simulink model "Pravahan_Powertrain_Powertrnblkset"  (R2023a)
settings: Solver=VariableStepAuto  StartTime=0.0  StopTime=5856  RelTol=1e-3
model workspace (MAT data in the model file):
  RPM = [0; 500; 500; 500; 500; 1000; 2000; 3000; 4000; 3000; 3000; 3000; 3000; 3300; 3300; 3300; 3000; 3000; 3000; 3000; 3000; 3500; 3500; 3500; 3500; 3000; 3000; 3000; 2500; 2000; 0; 0; 500; 1000; 2000; 3000; 4000; 3000; 3000; 3000; 3000; 3300; 3300; 3300; 3000; 3000; 3000; 3000; 3000; 3500; 3500; 3500; 3500; 3000; 3000; 3000; 3000; 3000; 3000; 2500; 2000; 0]
  Time = [0; 96; 192; 288; 384; 480; 576; 672; 768; 864; 960; 1056; 1152; 1248; 1344; 1440; 1536; 1632; 1728; 1824; 1920; 2016; 2112; 2208; 2304; 2400; 2496; 2592; 2688; 2784; 2880; 2976; 3072; 3168; 3264; 3360; 3456; 3552; 3648; 3744; 3840; 3936; 4032; 4128; 4224; 4320; 4416; 4512; 4608; 4704; 4800; 4896; 4992; 5088; 5184; 5280; 5376; 5472; 5568; 5664; 5760; 5856]
libraries: autolibrcnetworksystem x1, autolibmappedmotor x1
settings Model: Creator=Abhinandan  LastModifiedBy=Abhinandan

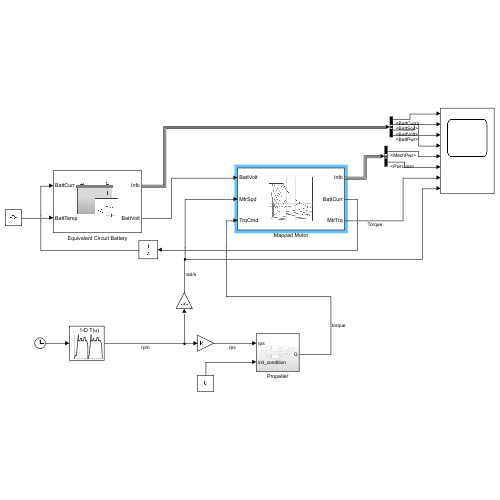
[thumbnail: Simulink's stored preview of the top-level diagram]
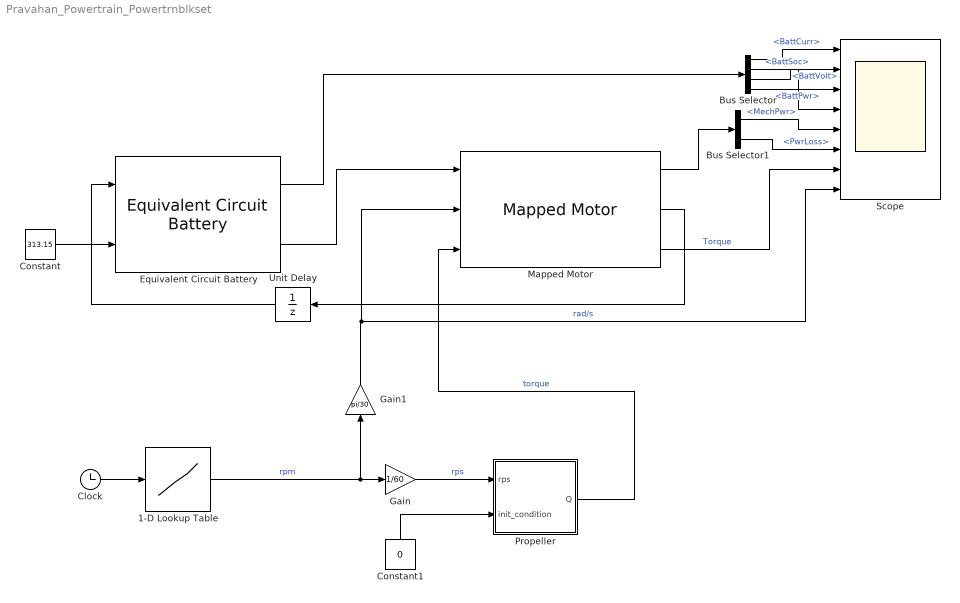
== system Pravahan_Powertrain_Powertrnblkset ==
  1-D Lookup Table : Lookup_n-D  NumberOfTableDimensions=1  BreakpointsForDimension1=Time  Table=RPM  InternalRulePriority=Speed  RndMeth=Simplest
  Bus Selector : BusSelector  OutputSignals=BattCurr,BattSoc,BattVolt,BattPwr
  Bus Selector1 : BusSelector  OutputSignals=MechPwr,PwrLoss
  Clock : Clock
  Constant : Constant  Value=313.15
  Constant1 : Constant  Value=0
  Equivalent Circuit Battery : autolibrcnetworksystem/Equivalent Circuit Battery  CapacityCtrl=Parameter  OutputVlt=Unfiltered  NumRC=1  Em=|  R0=|  SOC_BP=|  Temperature_BP=[293.15 313.15]  BattCap=[350 350]  BattCapInit=297.5  InitialCapVoltage=0  Tc=1/1000  Vinit=4.193  R1=|  C1=|  R2=|  C2=|  R3=|  C3=|  R4=|  C4=|  R5=|  C5=|  Vu=Inf  Vl=-Inf  RefBlkName='autolibrcnetworksystem/Equivalent Circuit Battery'
      Em=|
      | 62*[3.5042 3.5136;
      | 3.5573 3.5646;
      | 3.6009 3.6153;
      | 3.6393 3.6565;
      | 3.6742 3.6889;
      | 3.7121 3.7214;
      | 3.7937 3.8078;
      | 3.8753 3.8945;
      | 3.97 3.9859;
      | 4.0764 4.0821;
      | 4.1924 4.193]
      R0=|
      | (62/14)*[0.011448 0.0090006;
      | 0.011038 0.0089655;
      | 0.011281 0.0091261;
      | 0.011236 0.0091099;
      | 0.010959 0.008957;
      | 0.010714 0.0087969;
      | 0.010698 0.0089126;
      | 0.010712 0.0090517;
      | 0.010917 0.0090444;
      | 0.011304 0.0088992;
      | 0.011603 0.0089015
      | ]
      SOC_BP=|
      | [0
      | 0.1
      | 0.2
      | 0.3
      | 0.4
      | 0.5
      | 0.6
      | 0.7
      | 0.8
      | 0.9
      | 1]
      R1=|
      | (62/14)*[0.010342 0.0012244;
      | 0.0067316 0.0011396;
      | 0.0051156 0.0012661;
      | 0.0043447 0.0012265;
      | 0.0038826 0.0011163;
      | 0.0034226 0.0009968;
      | 0.003346 0.0011458;
      | 0.0033222 0.001345;
      | 0.0033201 0.0013091;
      | 0.0032886 0.0010986;
      | 0.0028114 0.0010309]
      C1=|
      | (14/62)*[2287.7 11897;
      | 6122 24515;
      | 18460 42098;
      | 20975 44453;
      | 15254 33098;
      | 10440 24492;
      | 13903 32975;
      | 16694 40007;
      | 15784 35937;
      | 12165 26430;
      | 9118 24795]
      R2=|
      | [0.010342 0.0012244;
      | 0.0067316 0.0011396;
      | 0.0051156 0.0012661;
      | 0.0043447 0.0012265;
      | 0.0038826 0.0011163;
      | 0.0034226 0.0009968;
      | 0.003346 0.0011458;
      | 0.0033222 0.001345;
      | 0.0033201 0.0013091;
      | 0.0032886 0.0010986;
      | 0.0028114 0.0010309]
      C2=|
      | [2287.7 11897;
      | 6122 24515;
      | 18460 42098;
      | 20975 44453;
      | 15254 33098;
      | 10440 24492;
      | 13903 32975;
      | 16694 40007;
      | 15784 35937;
      | 12165 26430;
      | 9118 24795]
      R3=|
      | [0.010342 0.0012244;
      | 0.0067316 0.0011396;
      | 0.0051156 0.0012661;
      | 0.0043447 0.0012265;
      | 0.0038826 0.0011163;
      | 0.0034226 0.0009968;
      | 0.003346 0.0011458;
      | 0.0033222 0.001345;
      | 0.0033201 0.0013091;
      | 0.0032886 0.0010986;
      | 0.0028114 0.0010309]
      C3=|
      | [2287.7 11897;
      | 6122 24515;
      | 18460 42098;
      | 20975 44453;
      | 15254 33098;
      | 10440 24492;
      | 13903 32975;
      | 16694 40007;
      | 15784 35937;
      | 12165 26430;
      | 9118 24795]
      R4=|
      | [0.010342 0.0012244;
      | 0.0067316 0.0011396;
      | 0.0051156 0.0012661;
      | 0.0043447 0.0012265;
      | 0.0038826 0.0011163;
      | 0.0034226 0.0009968;
      | 0.003346 0.0011458;
      | 0.0033222 0.001345;
      | 0.0033201 0.0013091;
      | 0.0032886 0.0010986;
      | 0.0028114 0.0010309]
      C4=|
      | [2287.7 11897;
      | 6122 24515;
      | 18460 42098;
      | 20975 44453;
      | 15254 33098;
      | 10440 24492;
      | 13903 32975;
      | 16694 40007;
      | 15784 35937;
      | 12165 26430;
      | 9118 24795]
      R5=|
      | [0.010342 0.0012244;
      | 0.0067316 0.0011396;
      | 0.0051156 0.0012661;
      | 0.0043447 0.0012265;
      | 0.0038826 0.0011163;
      | 0.0034226 0.0009968;
      | 0.003346 0.0011458;
      | 0.0033222 0.001345;
      | 0.0033201 0.0013091;
      | 0.0032886 0.0010986;
      | 0.0028114 0.0010309]
      C5=|
      | [2287.7 11897;
      | 6122 24515;
      | 18460 42098;
      | 20975 44453;
      | 15254 33098;
      | 10440 24492;
      | 13903 32975;
      | 16694 40007;
      | 15784 35937;
      | 12165 26430;
      | 9118 24795]
  Gain : Gain  Gain=1/60
  Gain1 : Gain  Gain=pi/30
  Mapped Motor : autolibmappedmotor/Mapped Motor  port_config=Speed  param_by=Maximum torque and power  w_t=[ 0 375 750 800 ]  T_t=[0.09 0.08 0.07 0]  torque_max=240  power_max=100000  Tc=0.02  param_loss=Tabulated efficiency data  eff=100  w_eff=375  T_eff=0.08  Piron=0  Pbase=0  w_eff_bp=[-300 -100 0 100 300]  T_eff_bp=[0 80 200 250]  Temp_eff_bp=[233.15 293.15 373.15]  losses_table=[1.49 1.67 2.21 3.10; 0.42 0.69 1.14 2.03; 0.06 0.24 0.78 1.68; 0.42 0.69 1.14 2.03; 1.49 1.67 2.21 3.10]  losses_table_3d=cat(3,[1.49 1.67 2.21 3.10; 0.42 0.69 1.14 2.03; 0.06 0.24 0.78 1.68; 0.42 0.69 1.14 2.03; 1.49 1.67 2.21 3.10],[1.49 1.67 2.21 3.10; 0.42 0.69 1.14 2.03; 0.06 0.24 0.78 1.68; 0.42 0.69 1.14 2.03; 1.49 1.67 2.21 3.10],[1.49 1.67 2.21 3.10; 0.42 0.69 1.14 2.03; 0.06 0.24 0.78 1.68; 0.42 0.69 1.14 2.03; 1.49 1.67 2.21 3.10])  efficiency_table=[94 94 94 94; 94 94 94 94; 94 94 94 94; 94 94 94 94; 94 94 94 94]  efficiency_table_3d=cat(3,[95 95 95 95; 95 95 95 95; 95 95 95 95; 95 95 95 95; 95 95 95 95],[95 95 95 95; 95 95 95 95; 95 95 95 95; 95 95 95 95; 95 95 95 95],[95 95 95 95; 95 95 95 95; 95 95 95 95; 95 95 95 95; 95 95 95 95])  J=5e-6  b=1e-5  omega_o=0  T_t_extended=[0 0.07 0.08 0.09 0.08 0.07 0]  w_t_extended=[-800 -750 -375 0 375 750 800]  KLossIron=0  KLossCopper=0  x_w_eff_vec=[-300 -100 0 100 300]  x_T_eff_vec=[-250 -200 -80 0 80 200 250]  x_tmp_eff_vec=[-0.09 -0.06 -0.03 0 0.03 0.06 0.09]  x_losses_mat=[4787.23404255319 3829.78723404255 1531.91489361702 0 1440 3600 4500;1595.74468085106 1276.59574468085 510.63829787234 0 480 1200 1500;0 0 0 0 0 0 0;1500 1200 480 0 510.63829787234 1276.59574468085 1595.74468085106;4500 3600 1440 0 1531.91489361702 3829.78723404255 4787.23404255319]  x_losses_mat_3d=[37.8947368421052 25.2631578947368 12.6315789473684 0 12 24 36;18.9473684210526 12.6315789473684 6.3157894736842 0 5.99999999999999 12 18;0 0 0 0 0 0 0;18 12 5.99999999999999 0 6.3157894736842 12.6315789473684 18.9473684210526;36 24 12 0 12.6315789473684 25.2631578947368 37.8947368421052]  CalLossMapData={}  CalLossWithTempMapData={}  aMode=1  RefBlkName='autolibmappedmotor/Mapped Motor'
      settings: LibrarySourceBlock=autolibemachines/Mapped Motor
  Propeller : Subsystem
  Scope : Scope  NumInputPorts=8
  Unit Delay : UnitDelay  SampleTime=-1  HasFrameUpgradeWarning=on
  wires:
  Equivalent Circuit Battery/2 -> Mapped Motor/1
  Equivalent Circuit Battery/1 -> Bus Selector/1
  Mapped Motor/2 -> Unit Delay/1
  Mapped Motor/1 -> Bus Selector1/1
  Constant/1 -> Equivalent Circuit Battery/2
  Bus Selector/1 -> Scope/1  "<BattCurr>"
  Bus Selector/2 -> Scope/4  "<BattSoc>"
  Bus Selector/3 -> Scope/2  "<BattVolt>"
  Bus Selector/4 -> Scope/3  "<BattPwr>"
  Bus Selector1/1 -> Scope/5  "<MechPwr>"
  Bus Selector1/2 -> Scope/6  "<PwrLoss>"
  Mapped Motor/3 -> Scope/7  "Torque"
  1-D Lookup Table/1 -> Gain/1, Gain1/1  "rpm"
  Propeller/1(Q) -> Mapped Motor/3  "torque"
  Gain/1 -> Propeller/1(rps)  "rps"
  Constant1/1 -> Propeller/2(init_condition)
  Gain1/1 -> Mapped Motor/2, Scope/8  "rad/s"
  Clock/1 -> 1-D Lookup Table/1
  Unit Delay/1 -> Equivalent Circuit Battery/1

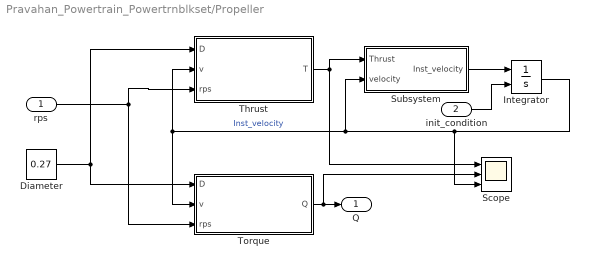
== system Pravahan_Powertrain_Powertrnblkset/Propeller ==
  rps : Inport
  init_condition : Inport  Port=2
  Diameter : Constant  Value=0.27
  Integrator : Integrator  InitialConditionSource=external
  Scope : Scope  NumInputPorts=3
  Subsystem : Subsystem
  Thrust : Subsystem
  Torque : Subsystem
  Q : Outport
  wires:
  Diameter/1 -> Torque/1(D), Thrust/1(D)
  rps/1 -> Torque/3(rps), Thrust/3(rps)
  Thrust/1(T) -> Scope/1, Subsystem/1(Thrust)
  Torque/1(Q) -> Scope/2, Q/1
  Integrator/1 -> Scope/3, Subsystem/2(velocity), Torque/2(v), Thrust/2(v)  "Inst_velocity"
  Subsystem/1(Inst_velocity) -> Integrator/1
  init_condition/1 -> Integrator/2

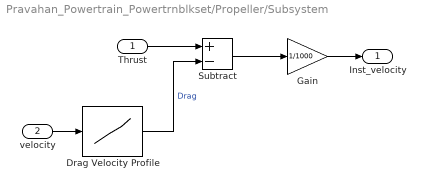
== system Pravahan_Powertrain_Powertrnblkset/Propeller/Subsystem ==
  Thrust : Inport
  velocity : Inport  Port=2
  Drag Velocity Profile : Lookup_n-D  NumberOfTableDimensions=1  BreakpointsForDimension1=[0 2.338181818 4.676363636 7.014545455 8.692839942 8.848719191 11.69090909 14.02909091 16.36727273 18.70545455 21.04363636]  Table=[0.1 2401.65157 3164.117316 3385.663625 3683.299572 1921.181996 1667.962675 1568.170036 1832.926016 1978.032659 2280.974598]  InternalRulePriority=Speed  RndMeth=Simplest
  Gain : Gain  Gain=1/1000
  Subtract : Sum  Inputs=+-
  Inst_velocity : Outport
  wires:
  Thrust/1 -> Subtract/1
  Drag Velocity Profile/1 -> Subtract/2  "Drag"
  Subtract/1 -> Gain/1
  velocity/1 -> Drag Velocity Profile/1
  Gain/1 -> Inst_velocity/1

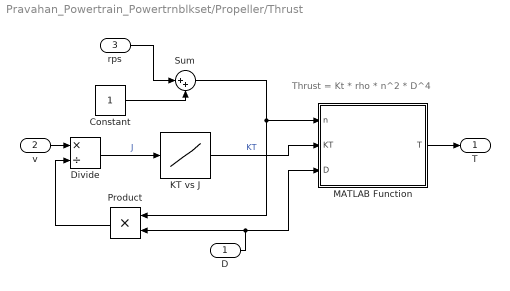
== system Pravahan_Powertrain_Powertrnblkset/Propeller/Thrust ==
  note: Thrust = Kt * rho * n^2 * D^4
  D : Inport
  v : Inport  Port=2
  rps : Inport  Port=3
  Constant : Constant
  Divide : Product  Inputs=*/
  KT vs J : Lookup_n-D  NumberOfTableDimensions=1  BreakpointsForDimension1=[0.0014;0.018198;0.034996;0.053193;0.074191;0.095188;0.109186;0.130184;0.151181;0.172178;0.195976;0.214173;0.23937;0.253368;0.274366;0.295363;0.31916;0.337358;0.354156;0.376553;0.393351;0.411549;0.432546;0.453543;0.473141;0.491339;0.512336;0.533333;0.550131;0.571129;0.589326;0.610324;0.635521;0.652318;0.676115;0.697113;0.72231;0.750306;0.774103;0.7993;0.827297;0.851094;0.869291;0.894488;0.925284;0.953281;0.974278;0.998075;1.019073;1.04147;1.065267;1.093263]  Table=[0.591807;0.582718;0.576664;0.564542;0.55394;0.546373;0.537281;0.531231;0.519112;0.508509;0.496392;0.481235;0.473672;0.466098;0.453978;0.443376;0.431259;0.420654;0.413082;0.397929;0.387323;0.378236;0.367633;0.352479;0.34491;0.332788;0.322185;0.310066;0.296425;0.28734;0.276735;0.264615;0.254017;0.241893;0.228259;0.216139;0.200989;0.185841;0.170689;0.155538;0.144942;0.128273;0.114633;0.102518;0.087372;0.072224;0.061622;0.049505;0.03435;0.026784;0.016185;0.001037]  InterpMethod=Cubic spline
  MATLAB Function : MATLAB Function  TreatAsAtomicUnit=on
  Product : Product
  Sum : Sum  Inputs=|++
  T : Outport
  wires:
  Sum/1 -> Product/1, MATLAB Function/1(n)
  D/1 -> Product/2, MATLAB Function/3(D)
  v/1 -> Divide/1
  Product/1 -> Divide/2
  Divide/1 -> KT vs J/1  "J"
  KT vs J/1 -> MATLAB Function/2(KT)  "KT"
  MATLAB Function/1(T) -> T/1
  rps/1 -> Sum/1
  Constant/1 -> Sum/2

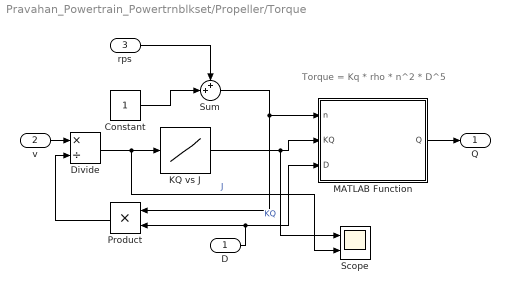
== system Pravahan_Powertrain_Powertrnblkset/Propeller/Torque ==
  note: Torque = Kq * rho * n^2 * D^5
  D : Inport
  v : Inport  Port=2
  rps : Inport  Port=3
  Constant : Constant
  Divide : Product  Inputs=*/
  KQ vs J : Lookup_n-D  NumberOfTableDimensions=1  BreakpointsForDimension1=[0;0.018198;0.039195;0.065792;0.088189;0.111986;0.135783;0.165179;0.188976;0.209974;0.230971;0.261767;0.286964;0.31776;0.338758;0.363955;0.384952;0.410149;0.433946;0.454943;0.47874;0.506737;0.527734;0.548731;0.566929;0.592126;0.620122;0.653718;0.678915;0.706912;0.734908;0.765704;0.7979;0.821697;0.849694;0.874891;0.895888;0.921085;0.940682;0.965879;0.993876;1.019073;1.04287;1.073666;1.096063;1.115661;1.143657;1.164654;1.190833]  Table=[0.096049;0.095151;0.093647;0.092147;0.091252;0.088535;0.087641;0.085232;0.08373;0.081619;0.080115;0.078618;0.07651;0.074102;0.07199;0.069577;0.068074;0.065661;0.063552;0.06144;0.059634;0.057528;0.056024;0.053912;0.051495;0.049994;0.046976;0.044874;0.042461;0.040355;0.037337;0.034928;0.032825;0.030412;0.028305;0.026805;0.024389;0.02228;0.020776;0.018971;0.016865;0.015364;0.013862;0.011758;0.010255;0.008751;0.005732;0.003317;0]
  MATLAB Function : MATLAB Function  TreatAsAtomicUnit=on
  Product : Product
  Scope : Scope  NumInputPorts=2
  Sum : Sum  Inputs=++|
  Q : Outport
  wires:
  MATLAB Function/1(Q) -> Q/1
  D/1 -> Product/2, MATLAB Function/3(D)
  Divide/1 -> Scope/2, KQ vs J/1  "J"
  v/1 -> Divide/1
  KQ vs J/1 -> Scope/1, MATLAB Function/2(KQ)  "KQ"
  Product/1 -> Divide/2
  Sum/1 -> Product/1, MATLAB Function/1(n)
  rps/1 -> Sum/1
  Constant/1 -> Sum/2

== matlab function Pravahan_Powertrain_Powertrnblkset/Propeller/Thrust/MATLAB Function ==
  data: n input; T output; KT input; D input
function T = fcn(n,KT,D)
    rho = 997;
    for i = length(n)
        T = KT * rho * n(i)^2 * D^4;
    end
end

== matlab function Pravahan_Powertrain_Powertrnblkset/Propeller/Torque/MATLAB Function ==
  data: n input; Q output; KQ input; D input
function Q = fcn(n,KQ,D)
    rho = 997;
    for i = length(n)
        Q = KQ * rho * n(i)^2 * D^5;
    end
end
